simulink model "KITTdynamics2"  (R2015b)
settings: Solver=VariableStepAuto  StartTime=0.0  StopTime=10  MaxStep=0.01  RelTol=1e-3
values from neighbouring files (symbols this model uses):
  c = 13    [KITTparameters2.m]
  Fa = 5    [KITTparameters2.m]
  Fd = 0.4    [KITTparameters2.m]
  m = 3    [KITTparameters2.m]
settings Model: Creator=Joran  LastModifiedBy=Mrklein
settings DataIOCC: SaveFinalState=on  SaveFormat=StructureWithTime  SaveState=on
settings DebuggingCC: MaxConsecutiveZCsMsg=none

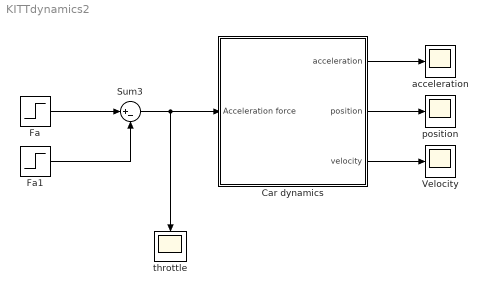
== system KITTdynamics2 ==
  "Car dynamics " : Subsystem
  Fa : Step  After=Fa  SampleTime=0
  Fa1 : Step  Time=6  After=Fa  SampleTime=0
  Sum3 : Sum  Inputs=|+-
  "Velocity " : Scope
  acceleration : Scope
  position : Scope
  throttle : Scope
  wires:
  Fa/1 -> Sum3/1
  Fa1/1 -> Sum3/2
  Sum3/1 -> throttle/1, "Car dynamics "/1(Acceleration force)
  "Car dynamics "/1(acceleration) -> acceleration/1
  "Car dynamics "/2("position ") -> position/1
  "Car dynamics "/3(velocity) -> "Velocity "/1

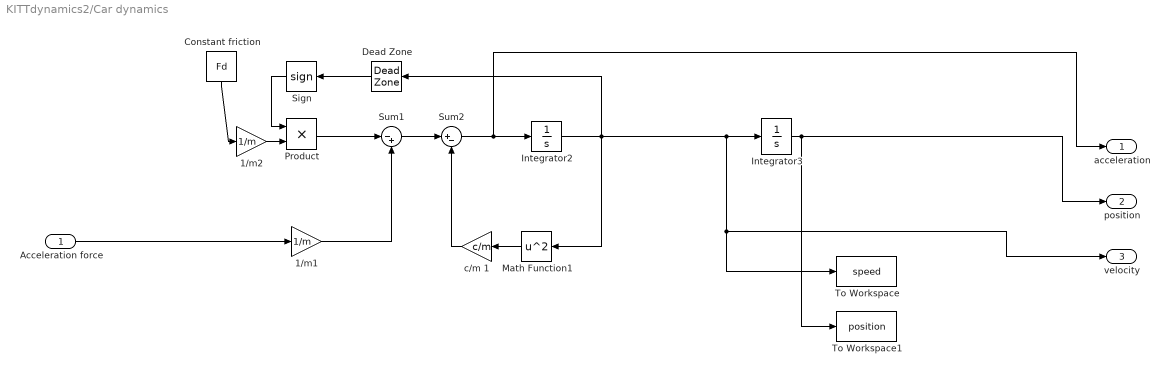
== system KITTdynamics2/Car dynamics  ==
  Acceleration force : Inport
  1/m1 : Gain  Gain=1/m
  1/m2 : Gain  Gain=1/m
  "Constant friction " : Constant  Value=Fd
  Dead Zone : DeadZone  LowerValue=-0.01  UpperValue=0.01  SaturateOnIntegerOverflow=on
  Integrator2 : Integrator
  Integrator3 : Integrator
  Math Function1 : Math  Operator=square  SaturateOnIntegerOverflow=on
  Product : Product
  Sign : Signum
  Sum1 : Sum  Inputs=|-+
  Sum2 : Sum  Inputs=|+-
  To Workspace : ToWorkspace  VariableName=speed  SaveFormat=Timeseries  SampleTime=-1
  To Workspace1 : ToWorkspace  VariableName=position  SaveFormat=Timeseries  SampleTime=-1
  c/m 1 : Gain  Gain=c/m
  acceleration : Outport
  "position " : Outport  Port=2
  velocity : Outport  Port=3
  wires:
  1/m2/1 -> Product/2
  Math Function1/1 -> c/m 1/1
  c/m 1/1 -> Sum2/2
  Integrator3/1 -> "position "/1, To Workspace1/1
  Integrator2/1 -> Math Function1/1, Dead Zone/1, velocity/1, To Workspace/1, Integrator3/1
  1/m1/1 -> Sum1/2
  "Constant friction "/1 -> 1/m2/1
  Product/1 -> Sum1/1
  Sign/1 -> Product/1
  Sum2/1 -> acceleration/1, Integrator2/1
  Sum1/1 -> Sum2/1
  Dead Zone/1 -> Sign/1
  Acceleration force/1 -> 1/m1/1
